simulink model "threeSurfaceThreeTether_th"  (R2018b)
settings: Solver=VariableStepAuto  StartTime=0.0  StopTime=0  RelTol=1e-3
undefined symbols (not defined in the file): ailDefl, elevDefl, mass, rudDefl, thr1TenVec, thr2TenVec, thr3TenVec, vWindVec
libraries: threeSurfaceThreeTether_cl x1
settings Model: Creator=mcobb  LastModifiedBy=mcobb

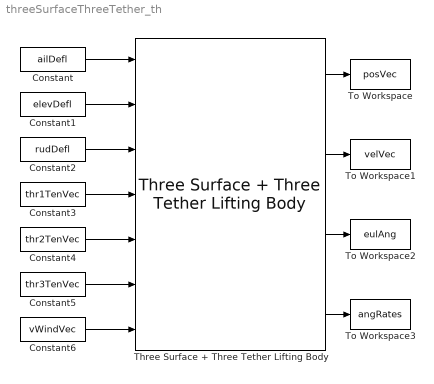
== system threeSurfaceThreeTether_th ==
  Constant : Constant  Value=ailDefl
  Constant1 : Constant  Value=elevDefl
  Constant2 : Constant  Value=rudDefl
  Constant3 : Constant  Value=thr1TenVec
  Constant4 : Constant  Value=thr2TenVec
  Constant5 : Constant  Value=thr3TenVec
  Constant6 : Constant  Value=vWindVec
  Three Surface + Three Tether Lifting Body : threeSurfaceThreeTether_cl/Three Surface + Three Tether Lifting Body  rho=rho  vol=vol  grav=grav  thr1PosVec=thr1Pt  thr2PosVec=thr2Pt  thr3PosVec=thr3Pt  turb1Pos=0  turb2Pos=0  turbDiam=0  turbCp=0  turbCd=0  CB2CMVec=cm2cbVec  m=mass  inertiaMatrix=intertiaMatrix  initPos=initPos  initVel=initVel  initEulerAngles=initEul  initAngRates=initEulRate  hStabWingAeroCentVec=hStabAC  hStabRotVec=hStabRotVec  hStabChordVec=hStabChord  hStabRefArea=hStabRefArea  hStabLiftCoeffFitParams=hStabLiftCoeffFitParams  hStabDragCoeffFitParams=hStabDragCoeffFitParams  vStabWingAeroCentVec=vStabAC  vStabRotVec=vStabRotVec  vStabChordVec=vStabChord  vStabRefArea=vStabRefArea  vStabLiftCoeffFitParams=vStabLiftCoeffFitParams  vStabDragCoeffFitParams=vStabDragCoeffFitParams  prtWingAeroCentVec=prtAC  prtRotVec=prtRotVec  prtChordVec=prtChord  prtRefArea=prtRefArea  prtLiftCoeffFitParams=prtLiftCoeffFitParams  prtDragCoeffFitParams=prtDragCoeffFitParams  sbdWingAeroCentVec=sbdAC  sbdRotVec=sbdRotVec  sbdChordVec=sbdChord  sbdRefArea=sbdRefArea  sbdLiftCoeffFitParams=sbdLiftCoeffFitParams  sbdDragCoeffFitParams=sbdDragCoeffFitParams
  To Workspace : ToWorkspace  VariableName=posVec  SaveFormat=Timeseries  SampleTime=-1
  To Workspace1 : ToWorkspace  VariableName=velVec  SaveFormat=Timeseries  SampleTime=-1
  To Workspace2 : ToWorkspace  VariableName=eulAng  SaveFormat=Timeseries  SampleTime=-1
  To Workspace3 : ToWorkspace  VariableName=angRates  SaveFormat=Timeseries  SampleTime=-1
  wires:
  Constant/1 -> Three Surface + Three Tether Lifting Body/1
  Constant2/1 -> Three Surface + Three Tether Lifting Body/3
  Constant1/1 -> Three Surface + Three Tether Lifting Body/2
  Constant3/1 -> Three Surface + Three Tether Lifting Body/4
  Constant4/1 -> Three Surface + Three Tether Lifting Body/5
  Constant5/1 -> Three Surface + Three Tether Lifting Body/6
  Constant6/1 -> Three Surface + Three Tether Lifting Body/7
  Three Surface + Three Tether Lifting Body/1 -> To Workspace/1
  Three Surface + Three Tether Lifting Body/2 -> To Workspace1/1
  Three Surface + Three Tether Lifting Body/3 -> To Workspace2/1
  Three Surface + Three Tether Lifting Body/4 -> To Workspace3/1
